simulink model "L02_TrafficLightController"  (R2021a)
settings: Solver=FixedStepDiscrete  StartTime=0.0  StopTime=120.0  FixedStep=0.1  RelTol=1e-3
settings Model: EnablePacing=on  PacingRate=2  Creator=ncleju  LastModifiedBy=ncleju

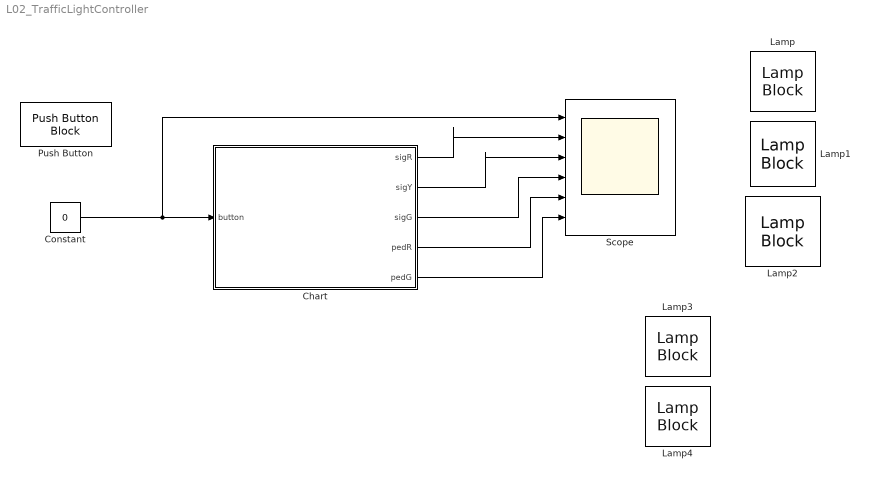
== system L02_TrafficLightController ==
  Chart : Stateflow chart  TreatAsAtomicUnit=on
  Constant : Constant  Value=0
  Lamp{,1..4} (5 alike) : LampBlock
  Push Button : PushButtonBlock
  Scope : Scope  NumInputPorts=6
  wires:
  Constant/1 -> Scope/1, Chart/1(button)
  Chart/1(sigR) -> Scope/2
  Chart/2(sigY) -> Scope/3
  Chart/3(sigG) -> Scope/4
  Chart/4(pedR) -> Scope/5
  Chart/5(pedG) -> Scope/6

== stateflow chart L02_TrafficLightController/Chart ==
  state RED
    entry:
    sigR=true;
    sigY=false;
    sigG=false;
    pedR=false;
    state A
      en: pedG=true;
    state B
      en: pedG=false;
    state C
      en: pedG=true;
    (default) -> A
    B -> C : [after(0.5,sec)]
    A -> B : [after(22,sec)]
    C -> B : [after(0.5,sec)]
  state GREEN
    entry:
    sigR=false;
    sigY=false;
    sigG=true;
    pedR=true;
    pedG=false;
  state GREEN_WAIT
  state YELLOW
    entry:
    sigR=false;
    %  sigY=true;
    sigG=false;
    pedR=true;
    pedG=false;
    state YELLOW_ON
      en: sigY=true;
    state YELLOW_OFF
      en: sigY=false;
    (default) -> YELLOW_ON
    YELLOW_ON -> YELLOW_OFF : [after(0.5,sec)]
    YELLOW_OFF -> YELLOW_ON : [after(0.5,sec)]
  (default) -> RED
  RED -> GREEN : [after(300, tick)]
      | {count=0;}
  GREEN -> GREEN [order 3] : [after(1,sec)]
      | {count = count+1;}
  GREEN -> GREEN_WAIT [order 2] : %[button == true && after(60, sec)==false]
      | [button == true]
  YELLOW -> RED : [after(5, sec)]
  GREEN -> YELLOW [order 1] : [button == true && count >=60]
  GREEN_WAIT -> YELLOW : [after(60 - count, sec)]
      | %after(60 - duration(buton == true,sec), sec)
  data: button input; sigR output; sigY output; sigG output; count local; pedR output; pedG output
